simulink model "SobelVHDL_Creation"  (R2024a)
settings: Solver=VariableStepAuto  StartTime=0.0  StopTime=10.0  RelTol=1e-3
libraries: dspsigops x1, visionhdlio x1, visionsources x1
settings Model: Creator=obb2733  LastModifiedBy=obb2733

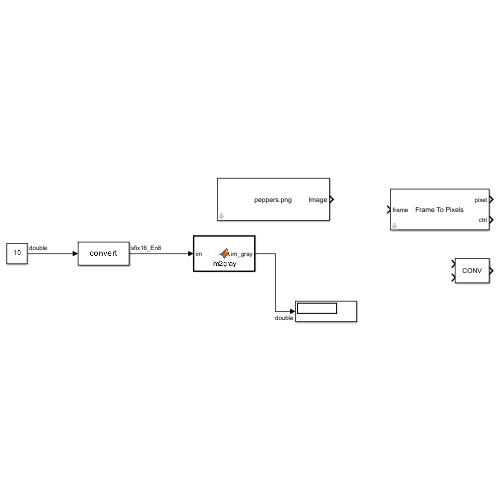
[thumbnail: Simulink's stored preview of the top-level diagram]
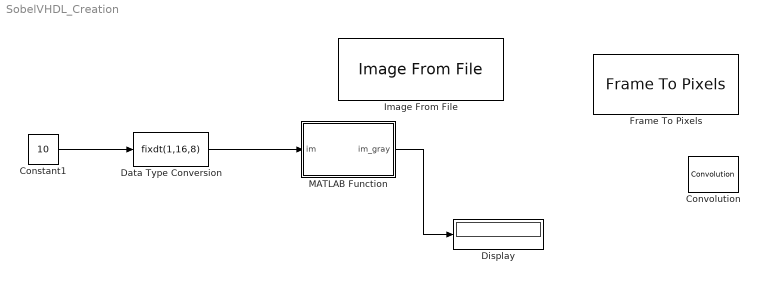
== system SobelVHDL_Creation ==
  Constant1 : Constant  Value=10  OutDataTypeStr=double
  Convolution : dspsigops/Convolution  domain=Time  roundingMode=Floor  overflowMode=off  outputDataTypeStr=Inherit: Same as accumulator  outputMin=[]  outputMax=[]  outputLastDataTypeStr=Inherit: Same as accumulator
  Data Type Conversion : DataTypeConversion  OutDataTypeStr=fixdt(1,16,8)  SaturateOnIntegerOverflow=off  RndMeth=Floor
  Display : Display
  Frame To Pixels : visionhdlio/Frame To Pixels  NumComponents=1  NumPixels=1  VideoFormat=1080p  ActivePixelsPerLine=1920  ActiveVideoLines=1080  TotalPixelsPerLine=2200  TotalVideoLines=1125  StartingActiveLine=42  FrontPorch=88  SampleTime=0  VideoFormatCache=1080p  ActivePixelsPerLineCache=32  ActiveVideoLinesCache=18  TotalPixelsPerLineCache=42  TotalVideoLinesCache=28  StartingActiveLineCache=6  FrontPorchCache=5
  Image From File : visionsources/Image From File  Tag=vipblks_nd  FileName=peppers.png  Ts=inf  imagePorts=One multidimensional signal  OutPortLabels=R|G|B  ImageDataType=Inherit from input image  sdImageDataType=uint(8)  Signed=on  WordLength=16  FractionLengthMode=User-defined  FractionLength=15
  MATLAB Function : MATLAB Function  TreatAsAtomicUnit=on
  wires:
  Constant1/1 -> Data Type Conversion/1
  Data Type Conversion/1 -> MATLAB Function/1(im)
  MATLAB Function/1(im_gray) -> Display/1

== matlab function SobelVHDL_Creation/MATLAB Function ==
  data: im input; im_gray output
function im_gray = im2gray(im)

% Apply Sobel Filter
im_gray = (0.2989 * double(im(:,:,1)) + 0.5870 * double(im(:,:,2)) + 0.1140 * double(im(:,:,3)))/255;
